simulink model "fig7_73ol"  (Simulink 4.00)
settings: Solver=ode23  StartTime=0.0  StopTime=300.0  RelTol=1e-6
settings Model: LastModifiedBy=abbas  LimitDataPoints=off  ExtModeTrigMode=oneshot  ExtModeArmWhenConnect=off  BlockReductionOpt=off

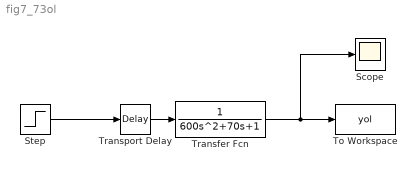
== system fig7_73ol ==
  Scope : Scope
      settings: TimeRange=auto  YMin=-5  YMax=5  SaveToWorkspace=off  SaveName=ScopeData  LimitDataPoints=on  MaxDataPoints=5000
  Step : Step  Time=1  Before=0  After=1  SampleTime=0
  To Workspace : ToWorkspace  VariableName=yol  SampleTime=-1  SaveFormat=Array
  Transfer Fcn : TransferFcn  Numerator=[1]  Denominator=[600 70 1]  Realization=auto  AbsoluteTolerance=auto
  Transport Delay : TransportDelay  DelayTime=5  InitialInput=0  BufferSize=1024  PadeOrder=0
  wires:
  Transport Delay/1 -> Transfer Fcn/1
  Transfer Fcn/1 -> To Workspace/1, Scope/1
  Step/1 -> Transport Delay/1
